simulink model "new_lv_try2"  (Simulink 7.1)
settings: Solver=ode3  StartTime=0.0  StopTime=1000  FixedStep=0.01  RelTol=1e-3
values from neighbouring files (symbols this model uses):
  Jem = 90    [lv_cankaofile.m]    (also in lv_demofile.m = 97.5; lv_demofile1.m = 97.5; lv_demofile2.m = 97.5; lv_demofile3.m = 97.5)
  Jwt = 9e7    (= 90000000)    [lv_cankaofile.m]    (also in lv_demofile.m = 3275300; lv_demofile1.m = 3275300; lv_demofile2.m = 3275300; lv_demofile3.m = 3275300)
  K = 83    [lv_cankaofile.m]    (also in lv_demofile.m; lv_demofile1.m = 75.76; lv_demofile2.m; lv_demofile3.m = 75.76)
  R = 40    [lv_cankaofile.m]    (also in lv_demofile.m = 38.5; lv_demofile1.m = 38.75; lv_demofile2.m = 38.5; lv_demofile3.m = 38.5)
  ro_air = 1.225    [lv_cankaofile.m]    (also in lv_demofile.m = 1.2236; lv_demofile1.m; lv_demofile2.m = 1.2236; lv_demofile3.m)
libraries: DRlib x1
settings Model: Creator=lv  LastModifiedBy=lv

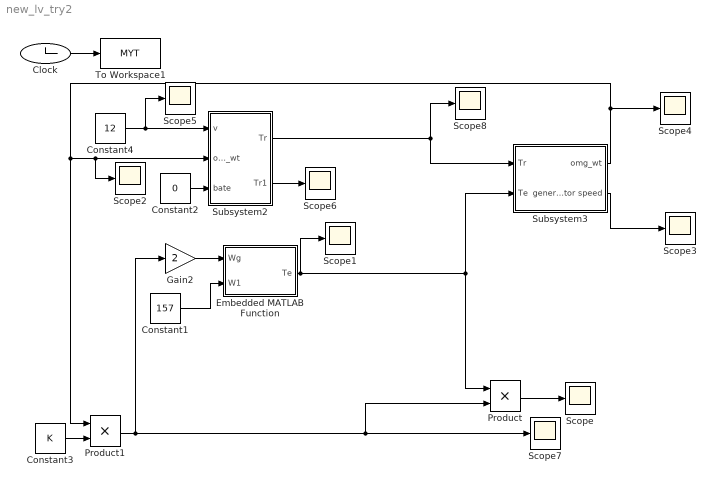
== system new_lv_try2 ==
  Clock : Clock
      settings: Decimation=10
  Constant1 : Constant  Value=157  OutDataType=sfix(16)  OutScaling=2^0
  Constant2 : Constant  Value=0  OutDataType=sfix(16)  OutScaling=2^0
  Constant3 : Constant  Value=K  OutDataType=sfix(16)  OutScaling=2^0
  Constant4 : Constant  Value=12  VectorParams1D=off  OutDataType=sfix(16)  OutScaling=2^0
  Embedded MATLAB Function : Stateflow chart
  Gain2 : Gain  Gain=2  ParameterDataType=sfix(16)  ParameterScaling=2^0  OutDataType=sfix(16)  OutScaling=2^0
  Product : Product  OutDataType=sfix(16)  OutScaling=2^0  RndMeth=Zero
  Product1 : Product  OutDataType=sfix(16)  OutScaling=2^0  RndMeth=Zero
  Scope{,1..8} (9 alike) : Scope
      Scope settings: TimeRange=200  YMin=1.01801e+006  YMax=1.01801e+006  SaveName=ScopeData9
      Scope1 settings: YMin=0  YMax=170000  SaveName=ScopeData13
      Scope2 settings: SaveName=ScopeData14
      Scope3 settings: YMin=74.6079  YMax=82.4613  SaveName=ScopeData15
      Scope4 settings: SaveName=ScopeData16
      Scope5 settings: SaveName=ScopeData17
      Scope6 settings: SaveName=ScopeData18
      Scope7 settings: YMin=277.719  YMax=306.953  SaveName=ScopeData19
      Scope8 settings: YMin=100000  YMax=700000  SaveName=ScopeData22
  Subsystem2 : Subsystem
  Subsystem3 : Subsystem
  To Workspace1 : ToWorkspace  VariableName=MYT  SampleTime=-1  SaveFormat=Array
  wires:
  Subsystem3/2(generator speed) -> Scope3/1
  Constant4/1 -> Subsystem2/1(v), Scope5/1
  Constant2/1 -> Subsystem2/3(bate)
  Subsystem3/1(omg_wt) -> Scope4/1, Subsystem2/2(omg_wt), Scope2/1, Product1/1
  Product/1 -> Scope/1
  Subsystem2/2(Tr1) -> Scope6/1
  Constant3/1 -> Product1/2
  Product1/1 -> Product/2, Scope7/1, Gain2/1
  Subsystem2/1(Tr) -> Scope8/1, Subsystem3/1(Tr)
  Embedded MATLAB Function/1(Te) -> Product/1, Subsystem3/2(Te), Scope1/1
  Clock/1 -> To Workspace1/1
  Constant1/1 -> Embedded MATLAB Function/2(W1)
  Gain2/1 -> Embedded MATLAB Function/1(Wg)

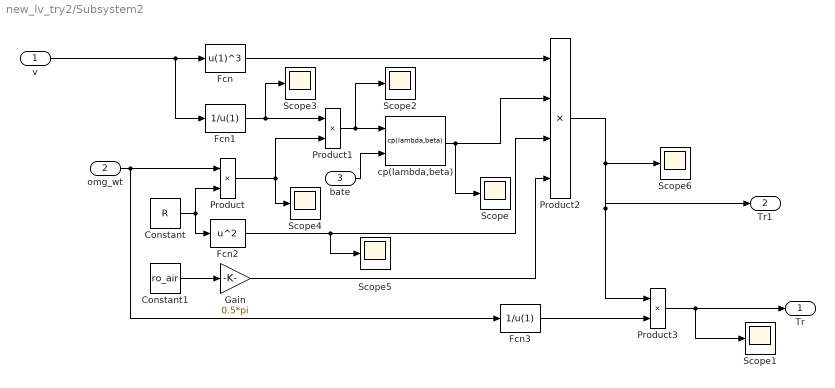
== system new_lv_try2/Subsystem2 ==
  v : Inport  OutDataType=sfix(16)  OutScaling=2^0
  omg_wt : Inport  Port=2  OutDataType=sfix(16)  OutScaling=2^0
  bate : Inport  Port=3  OutDataType=sfix(16)  OutScaling=2^0
  Constant : Constant  Value=R  OutDataType=sfix(16)  OutScaling=2^0
  Constant1 : Constant  Value=ro_air  OutDataType=sfix(16)  OutScaling=2^0
  Fcn : Fcn  Expr=u(1)^3
  Fcn1 : Fcn  Expr=1/u(1)
  Fcn2 : Fcn  Expr=u^2
  Fcn3 : Fcn  Expr=1/u(1)
  Gain : Gain  Gain=0.5*pi  ParameterDataType=sfix(16)  ParameterScaling=2^0  OutDataType=sfix(16)  OutScaling=2^0
  Product : Product  OutDataType=sfix(16)  OutScaling=2^0  RndMeth=Zero
  Product1 : Product  OutDataType=sfix(16)  OutScaling=2^0  RndMeth=Zero
  Product2 : Product  Inputs=4  OutDataType=sfix(16)  OutScaling=2^0  RndMeth=Zero
  Product3 : Product  OutDataType=sfix(16)  OutScaling=2^0  RndMeth=Zero
  Scope{,1..6} (7 alike) : Scope
      Scope settings: TimeRange=50  YMin=0.1772981595092024  YMax=0.2028981595092024  SaveName=ScopeData4
      Scope1 settings: TimeRange=20  YMin=-1500000  YMax=1500000
      Scope2 settings: SaveName=ScopeData6
      Scope3 settings: SaveName=ScopeData7
      Scope4 settings: SaveName=ScopeData8
      Scope5 settings: YMin=1426.48  YMax=1576.64  SaveName=ScopeData20
      Scope6 settings: TimeRange=20  YMin=-500000  YMax=5e+006  SaveName=ScopeData21
  cp(lambda,beta) : DRlib/Wind Generation/Wind Turbine/cp(lambda,beta)  SystemSampleTime=-1
  Tr : Outport  OutDataType=sfix(16)  OutScaling=2^0
  Tr1 : Outport  Port=2  OutDataType=sfix(16)  OutScaling=2^0
  wires:
  v/1 -> Fcn/1, Fcn1/1
  omg_wt/1 -> Product/1, Fcn3/1
  Constant/1 -> Product/2, Fcn2/1
  Fcn1/1 -> Product1/1, Scope3/1
  Product/1 -> Product1/2, Scope4/1
  Product1/1 -> Scope2/1, cp(lambda,beta)/1
  bate/1 -> cp(lambda,beta)/2
  Fcn/1 -> Product2/1
  cp(lambda,beta)/1 -> Scope/1, Product2/2
  Fcn2/1 -> Product2/3, Scope5/1
  Gain/1 -> Product2/4
  Constant1/1 -> Gain/1
  Product2/1 -> Scope6/1, Product3/1, Tr1/1
  Fcn3/1 -> Product3/2
  Product3/1 -> Scope1/1, Tr/1

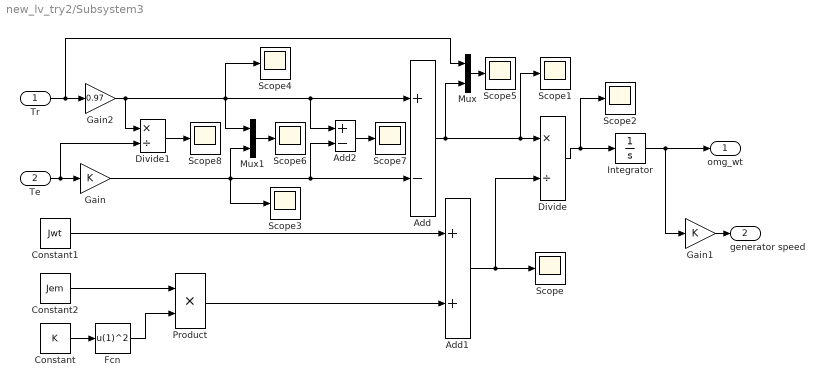
== system new_lv_try2/Subsystem3 ==
  Tr : Inport  OutDataType=sfix(16)  OutScaling=2^0
  Te : Inport  Port=2  OutDataType=sfix(16)  OutScaling=2^0
  Add : Sum  Inputs=+-  OutDataType=sfix(16)  OutScaling=2^-10
  Add1 : Sum  OutDataType=sfix(16)  OutScaling=2^-10
  Add2 : Sum  Inputs=+-  OutDataType=sfix(16)  OutScaling=2^-10
  Constant : Constant  Value=K  OutDataType=sfix(16)  OutScaling=2^0
  Constant1 : Constant  Value=Jwt  OutDataType=sfix(16)  OutScaling=2^0
  Constant2 : Constant  Value=Jem  OutDataType=sfix(16)  OutScaling=2^0
  Divide : Product  Inputs=*/  OutDataType=sfix(16)  OutScaling=2^-10
  Divide1 : Product  Inputs=*/  OutDataType=sfix(16)  OutScaling=2^-10
  Fcn : Fcn  Expr=u(1)^2
  Gain : Gain  Gain=K  ParameterDataType=sfix(16)  ParameterScaling=2^0  OutDataType=sfix(16)  OutScaling=2^0
  Gain1 : Gain  Gain=K  ParameterDataType=sfix(16)  ParameterScaling=2^0  OutDataType=sfix(16)  OutScaling=2^0
  Gain2 : Gain  Gain=0.97  ParameterDataType=sfix(16)  ParameterScaling=2^0  OutDataType=sfix(16)  OutScaling=2^0
  Integrator : Integrator  InitialCondition=1.9
  Mux : Mux  Inputs=2
  Mux1 : Mux  Inputs=2
  Product : Product  OutDataType=sfix(16)  OutScaling=2^0  RndMeth=Zero
  Scope{,1..8} (9 alike) : Scope
      Scope settings: SaveName=ScopeData5
      Scope1 settings: YMin=1.27737e-008  YMax=1.41183e-008  SaveName=ScopeData6
      Scope2 settings: SaveName=ScopeData7
      Scope3 settings: SaveName=ScopeData23
      Scope4 settings: SaveName=ScopeData24
      Scope5 settings: SaveName=ScopeData25
      Scope6 settings: TimeRange=100  YMin=213472  YMax=235942  SaveName=ScopeData3
      Scope7 settings: SaveName=ScopeData11
      Scope8 settings: YMin=75  YMax=145
  omg_wt : Outport  OutDataType=sfix(16)  OutScaling=2^0
  generator speed : Outport  Port=2  OutDataType=sfix(16)  OutScaling=2^0
  wires:
  Fcn/1 -> Product/2
  Constant/1 -> Fcn/1
  Te/1 -> Gain/1, Divide1/2
  Tr/1 -> Mux/1, Gain2/1
  Gain/1 -> Mux1/2, Add2/2, Add/2, Scope3/1
  Constant2/1 -> Product/1
  Constant1/1 -> Add1/1
  Product/1 -> Add1/2
  Add/1 -> Scope1/1, Divide/1, Mux/2
  Add1/1 -> Scope/1, Divide/2
  Divide/1 -> Scope2/1, Integrator/1
  Integrator/1 -> Gain1/1, omg_wt/1
  Gain1/1 -> generator speed/1
  Mux/1 -> Scope5/1
  Mux1/1 -> Scope6/1
  Gain2/1 -> Mux1/1, Scope4/1, Add/1, Add2/1, Divide1/1
  Add2/1 -> Scope7/1
  Divide1/1 -> Scope8/1

== matlab function Embedded MATLAB Function ==
  data: Wg input double; Te output double; W1 input double
function Te = fcn(Wg,W1)
%#eml
% This block supports the Embedded MATLAB subset.
% See the help menu for details. 

Te=6855.84/((Wg-W1)*((0.00169-0.813*0.0024*W1/(Wg-W1))^2+(0.03692+0.813*0.03759)^2));
%Te = 6855.84/((Wg-W1)*(0.00169-0.813*0.0024*W1/(Wg-W1))^2+(0.03692+0.813*0.03759)^2);
